simulink library "inp_BCKP"  (R2021b)
settings: Solver=VariableStepAuto  StartTime=0.0  StopTime=10.0  RelTol=1e-3
undefined symbols (not defined in the file): C_TASK_5MS_S, FALSE, KINP_AcoreReadyToSlp_flg_ovrdflg, KINP_AcoreReadyToSlp_flg_ovrdval, KINP_AllowMovThd_OTA_enum_ovrdflg, KINP_AllowMovThd_OTA_enum_ovrdval, KINP_APSAngleTarget_Deg_ovrdflg, KINP_APSAngleTarget_Deg_ovrdval, KINP_APSDecReq_mps2_ovrdflg, KINP_APSDecReq_mps2_ovrdval, KINP_APSDecReqA_flg_ovrdflg, KINP_APSDecReqA_flg_ovrdval, KINP_APSDFLL_cm_ovrdflg, KINP_APSDFLL_cm_ovrdval, KINP_APSDFLR_cm_ovrdflg, KINP_APSDFLR_cm_ovrdval, KINP_APSDRLL_cm_ovrdflg, KINP_APSDRLL_cm_ovrdval, KINP_APSDRLR_cm_ovrdflg, KINP_APSDRLR_cm_ovrdval, KINP_APSExitCondition_enum_ovrdflg, KINP_APSExitCondition_enum_ovrdval, KINP_APSHWVer_enum_ovrdflg, KINP_APSHWVer_enum_ovrdval, KINP_APSProgressPCT_pct_ovrdflg, KINP_APSProgressPCT_pct_ovrdval, KINP_APSPwrReq_enum_ovrdflg, KINP_APSPwrReq_enum_ovrdval, KINP_APSReq_enum_ovrdflg, KINP_APSReq_enum_ovrdval, KINP_APSRQDisplay_enum_ovrdflg, KINP_APSRQDisplay_enum_ovrdval, KINP_APSRqEPASCtrl_flg_ovrdflg, KINP_APSRqEPASCtrl_flg_ovrdval, KINP_APSShiftPosnReq_enum_ovrdval, KINP_APSShiftPosnReq_enum_ovrflg, KINP_APSSpeedCMD_kph_ovrdval, KINP_APSSpeedCMD_kph_ovrflg, KINP_APSStaSystem_enum_ovrdflg, KINP_APSStaSystem_enum_ovrdval, KINP_APSSWVer_enum_ovrdflg, KINP_APSSWVer_enum_ovrdval, KINP_APSVMCReqA_flg_ovrdval, KINP_APSVMCReqA_flg_ovrflg, KINP_APSVRqEPASCtrl_flg_ovrdflg, KINP_APSVRqEPASCtrl_flg_ovrdval, KINP_AuxBattVolmV_mV_ovrdflg, KINP_AuxBattVolmV_mV_ovrdval, KINP_BTConnectSta_enum_ovrdflg, KINP_BTConnectSta_enum_ovrdval, KINP_CAASSta_enum_ovrdflg, KINP_CAASSta_enum_ovrdval, KINP_CAASVMCReqA_flg_ovrdval, KINP_CAASVMCReqA_flg_ovrflg, KINP_CAN1BusOff_flg_ovrdflg, KINP_CAN1BusOff_flg_ovrdval, KINP_CAN2BusOff_flg_ovrdflg, KINP_CAN2BusOff_flg_ovrdval, KINP_CAN3BusOff_flg_ovrdflg, KINP_CAN3BusOff_flg_ovrdval ... (+158)
libraries: FVT_lib x144, hcu_lib x1
(part 3 of 8)

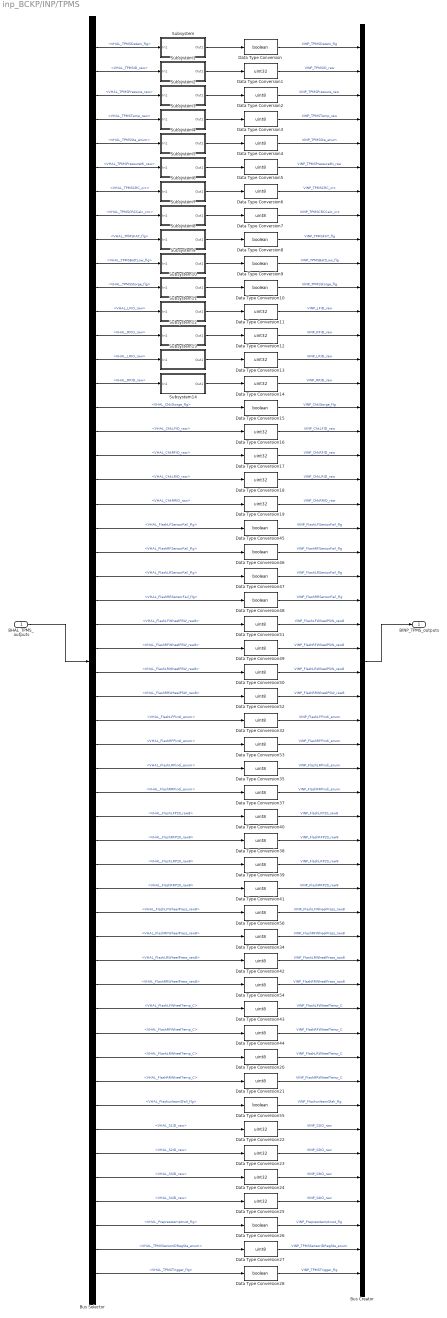
== system inp_BCKP/INP/TPMS ==
  BHAL_TPMS_outputs : Inport  OutDataTypeStr=Bus: BHAL_TPMS_outputs
  Bus Creator : BusCreator  Inputs=52  OutDataTypeStr=Bus: BINP_TPMS_outputs  NonVirtualBus=on
  Bus Selector : BusSelector  OutputSignals=VHAL_TPMSDataIn_flg,VHAL_TPMSID_raw,VHAL_TPMSPressure_raw,VHAL_TPMSTemp_raw,VHAL_TPMSSta_enum,VHAL_TPMSPressureMi_raw,VHAL_TPMSCRC_crc,VHAL_TPMSCRCCalc_crc,VHAL_TPMSFAT_flg,VHAL_TPMSBattLow_flg,VHAL_TPMSStorge_flg,VHAL_LFID_raw,VHAL_RFID_raw,VHAL_LRID_raw,VHAL_RRID_raw,VHAL_ChkStorge_flg,VHAL_ChkLFID_raw,VHAL_ChkRFID_raw,VHAL_ChkLRID_raw,VHAL_ChkRRID_raw,VHAL_FlashLFSensorFail_flg,VHAL_FlashRFSensorFail_flg,VHAL_FlashLRSensorFail_flg,VHAL_FlashRRSensorFail_flg,VHAL_FlashLFWheelPSW_raw8,VHAL_FlashRFWheelPSW_raw8,VHAL_FlashLRWheelPSW_raw8,VHAL_FlashRRWheelPSW_raw8,VHAL_FlashLFPindi_enum,VHAL_FlashRFPindi_enum,VHAL_FlashLRPindi_enum,VHAL_FlashRRPindi_enum,VHAL_FlashLFP20_raw8,VHAL_FlashRFP20_raw8,VHAL_FlashLRP20_raw8,VHAL_FlashRRP20_raw8,VHAL_FlashLFWheelPress_raw8,VHAL_FlashRFWheelPress_raw8,VHAL_FlashLRWheelPress_raw8,VHAL_FlashRRWheelPress_raw8,VHAL_FlashLFWheelTemp_C,VHAL_FlashRFWheelTemp_C,VHAL_FlashLRWheelTemp_C,VHAL_FlashRRWheelTemp_C,VHAL_FlashunlearnSfali_flg,VHAL_S1ID_raw,VHAL_S2ID_raw,VHAL_S3ID_raw,VHAL_S4ID_raw,VHAL_Prepresstemptrust_flg,VHAL_TPMSSensorIDRegSta_enum,VHAL_TPMSTrigger_flg
  Data Type Conversion{,8..10,15,26,28,45..48,55} (12 alike) : DataTypeConversion  OutDataTypeStr=boolean
  Data Type Conversion{1,11..14,16..19,22..25} (13 alike) : DataTypeConversion  OutDataTypeStr=uint32
  Data Type Conversion{2..7,20..21,27,32,34..35,37..44,49..54,56} (27 alike) : DataTypeConversion  OutDataTypeStr=uint8
  Subsystem : Subsystem
  Subsystem1 : Subsystem
  Subsystem10 : Subsystem
  Subsystem11 : Subsystem
  Subsystem12 : Subsystem
  Subsystem13 : Subsystem
  Subsystem14 : Subsystem
  Subsystem2 : Subsystem
  Subsystem3 : Subsystem
  Subsystem4 : Subsystem
  Subsystem5 : Subsystem
  Subsystem6 : Subsystem
  Subsystem7 : Subsystem
  Subsystem8 : Subsystem
  Subsystem9 : Subsystem
  BINP_TPMS_outputs : Outport  OutDataTypeStr=Bus: BINP_TPMS_outputs
  wires:
  Bus Selector/49 -> Data Type Conversion25/1  "<VHAL_S4ID_raw>"
  Bus Selector/48 -> Data Type Conversion24/1  "<VHAL_S3ID_raw>"
  Bus Selector/47 -> Data Type Conversion23/1  "<VHAL_S2ID_raw>"
  Bus Selector/46 -> Data Type Conversion22/1  "<VHAL_S1ID_raw>"
  Data Type Conversion25/1 -> Bus Creator/49  "VINP_S4ID_raw"
  Data Type Conversion24/1 -> Bus Creator/48  "VINP_S3ID_raw"
  Data Type Conversion23/1 -> Bus Creator/47  "VINP_S2ID_raw"
  Data Type Conversion22/1 -> Bus Creator/46  "VINP_S1ID_raw"
  Data Type Conversion21/1 -> Bus Creator/44  "VINP_FlashRRWheelTemp_C"
  Data Type Conversion20/1 -> Bus Creator/43  "VINP_FlashLRWheelTemp_C"
  Bus Selector/44 -> Data Type Conversion21/1  "<VHAL_FlashRRWheelTemp_C>"
  Bus Selector/43 -> Data Type Conversion20/1  "<VHAL_FlashLRWheelTemp_C>"
  Data Type Conversion55/1 -> Bus Creator/45  "VINP_FlashunlearnSfali_flg"
  Bus Selector/45 -> Data Type Conversion55/1  "<VHAL_FlashunlearnSfali_flg>"
  Data Type Conversion44/1 -> Bus Creator/42  "VINP_FlashRFWheelTemp_C"
  Bus Selector/42 -> Data Type Conversion44/1  "<VHAL_FlashRFWheelTemp_C>"
  Data Type Conversion43/1 -> Bus Creator/41  "VINP_FlashLFWheelTemp_C"
  Bus Selector/41 -> Data Type Conversion43/1  "<VHAL_FlashLFWheelTemp_C>"
  Data Type Conversion54/1 -> Bus Creator/40  "VINP_FlashRRWheelPress_raw8"
  Data Type Conversion42/1 -> Bus Creator/39  "VINP_FlashLRWheelPress_raw8"
  Bus Selector/40 -> Data Type Conversion54/1  "<VHAL_FlashRRWheelPress_raw8>"
  Bus Selector/39 -> Data Type Conversion42/1  "<VHAL_FlashLRWheelPress_raw8>"
  Data Type Conversion34/1 -> Bus Creator/38  "VINP_FlashRFWheelPress_raw8"
  Bus Selector/38 -> Data Type Conversion34/1  "<VHAL_FlashRFWheelPress_raw8>"
  Data Type Conversion56/1 -> Bus Creator/37  "VINP_FlashLFWheelPress_raw8"
  Bus Selector/37 -> Data Type Conversion56/1  "<VHAL_FlashLFWheelPress_raw8>"
  Data Type Conversion41/1 -> Bus Creator/36  "VINP_FlashRRP20_raw8"
  Bus Selector/36 -> Data Type Conversion41/1  "<VHAL_FlashRRP20_raw8>"
  Data Type Conversion39/1 -> Bus Creator/35  "VINP_FlashLRP20_raw8"
  Bus Selector/35 -> Data Type Conversion39/1  "<VHAL_FlashLRP20_raw8>"
  Data Type Conversion38/1 -> Bus Creator/34  "VINP_FlashRFP20_raw8"
  Bus Selector/34 -> Data Type Conversion38/1  "<VHAL_FlashRFP20_raw8>"
  Data Type Conversion40/1 -> Bus Creator/33  "VINP_FlashLFP20_raw8"
  Bus Selector/33 -> Data Type Conversion40/1  "<VHAL_FlashLFP20_raw8>"
  Data Type Conversion37/1 -> Bus Creator/32  "VINP_FlashRRPindi_enum"
  Bus Selector/32 -> Data Type Conversion37/1  "<VHAL_FlashRRPindi_enum>"
  Data Type Conversion35/1 -> Bus Creator/31  "VINP_FlashLRPindi_enum"
  Bus Selector/31 -> Data Type Conversion35/1  "<VHAL_FlashLRPindi_enum>"
  Data Type Conversion53/1 -> Bus Creator/30  "VINP_FlashRFPindi_enum"
  Bus Selector/30 -> Data Type Conversion53/1  "<VHAL_FlashRFPindi_enum>"
  Data Type Conversion32/1 -> Bus Creator/29  "VINP_FlashLFPindi_enum"
  Bus Selector/29 -> Data Type Conversion32/1  "<VHAL_FlashLFPindi_enum>"
  Data Type Conversion52/1 -> Bus Creator/28  "VINP_FlashRRWheelPSW_raw8"
  Bus Selector/28 -> Data Type Conversion52/1  "<VHAL_FlashRRWheelPSW_raw8>"
  Data Type Conversion50/1 -> Bus Creator/27  "VINP_FlashLRWheelPSW_raw8"
  Bus Selector/27 -> Data Type Conversion50/1  "<VHAL_FlashLRWheelPSW_raw8>"
  Data Type Conversion49/1 -> Bus Creator/26  "VINP_FlashRFWheelPSW_raw8"
  Bus Selector/26 -> Data Type Conversion49/1  "<VHAL_FlashRFWheelPSW_raw8>"
  Data Type Conversion51/1 -> Bus Creator/25  "VINP_FlashLFWheelPSW_raw8"
  Bus Selector/25 -> Data Type Conversion51/1  "<VHAL_FlashLFWheelPSW_raw8>"
  Data Type Conversion48/1 -> Bus Creator/24  "VINP_FlashRRSensorFail_flg"
  Bus Selector/24 -> Data Type Conversion48/1  "<VHAL_FlashRRSensorFail_flg>"
  Data Type Conversion47/1 -> Bus Creator/23  "VINP_FlashLRSensorFail_flg"
  Bus Selector/23 -> Data Type Conversion47/1  "<VHAL_FlashLRSensorFail_flg>"
  Data Type Conversion46/1 -> Bus Creator/22  "VINP_FlashRFSensorFail_flg"
  Bus Selector/22 -> Data Type Conversion46/1  "<VHAL_FlashRFSensorFail_flg>"
  Data Type Conversion45/1 -> Bus Creator/21  "VINP_FlashLFSensorFail_flg"
  Bus Selector/21 -> Data Type Conversion45/1  "<VHAL_FlashLFSensorFail_flg>"
  Data Type Conversion19/1 -> Bus Creator/20  "VINP_ChkRRID_raw"
  Data Type Conversion18/1 -> Bus Creator/19  "VINP_ChkLRID_raw"
  Data Type Conversion17/1 -> Bus Creator/18  "VINP_ChkRFID_raw"
  Data Type Conversion16/1 -> Bus Creator/17  "VINP_ChkLFID_raw"
  Data Type Conversion15/1 -> Bus Creator/16  "VINP_ChkStorge_flg"
  Bus Selector/20 -> Data Type Conversion19/1  "<VHAL_ChkRRID_raw>"
  Bus Selector/19 -> Data Type Conversion18/1  "<VHAL_ChkLRID_raw>"
  Bus Selector/18 -> Data Type Conversion17/1  "<VHAL_ChkRFID_raw>"
  Bus Selector/17 -> Data Type Conversion16/1  "<VHAL_ChkLFID_raw>"
  Bus Selector/16 -> Data Type Conversion15/1  "<VHAL_ChkStorge_flg>"
  Data Type Conversion14/1 -> Bus Creator/15  "VINP_RRID_raw"
  Data Type Conversion13/1 -> Bus Creator/14  "VINP_LRID_raw"
  Data Type Conversion12/1 -> Bus Creator/13  "VINP_RFID_raw"
  Data Type Conversion11/1 -> Bus Creator/12  "VINP_LFID_raw"
  Subsystem14/1(Out1) -> Data Type Conversion14/1
  Subsystem13/1(Out1) -> Data Type Conversion13/1
  Subsystem12/1(Out1) -> Data Type Conversion12/1
  Subsystem11/1(Out1) -> Data Type Conversion11/1
  Bus Selector/15 -> Subsystem14/1(In1)  "<VHAL_RRID_raw>"
  Bus Selector/14 -> Subsystem13/1(In1)  "<VHAL_LRID_raw>"
  Bus Selector/13 -> Subsystem12/1(In1)  "<VHAL_RFID_raw>"
  Bus Selector/12 -> Subsystem11/1(In1)  "<VHAL_LFID_raw>"
  Data Type Conversion10/1 -> Bus Creator/11  "VINP_TPMSStorge_flg"
  Subsystem10/1(Out1) -> Data Type Conversion10/1
  Bus Selector/11 -> Subsystem10/1(In1)  "<VHAL_TPMSStorge_flg>"
  Subsystem9/1(Out1) -> Data Type Conversion9/1
  Subsystem8/1(Out1) -> Data Type Conversion8/1
  Bus Selector/10 -> Subsystem9/1(In1)  "<VHAL_TPMSBattLow_flg>"
  Bus Selector/9 -> Subsystem8/1(In1)  "<VHAL_TPMSFAT_flg>"
  Data Type Conversion9/1 -> Bus Creator/10  "VINP_TPMSBattLow_flg"
  Data Type Conversion8/1 -> Bus Creator/9  "VINP_TPMSFAT_flg"
  Bus Creator/1 -> BINP_TPMS_outputs/1
  Data Type Conversion7/1 -> Bus Creator/8  "VINP_TPMSCRCCalc_crc"
  Data Type Conversion6/1 -> Bus Creator/7  "VINP_TPMSCRC_crc"
  Data Type Conversion5/1 -> Bus Creator/6  "VINP_TPMSPressureMi_raw"
  Data Type Conversion4/1 -> Bus Creator/5  "VINP_TPMSSta_enum"
  Data Type Conversion3/1 -> Bus Creator/4  "VINP_TPMSTemp_raw"
  Data Type Conversion2/1 -> Bus Creator/3  "VINP_TPMSPressure_raw"
  Data Type Conversion1/1 -> Bus Creator/2  "VINP_TPMSID_raw"
  Data Type Conversion/1 -> Bus Creator/1  "VINP_TPMSDataIn_flg"
  Subsystem7/1(Out1) -> Data Type Conversion7/1
  Subsystem6/1(Out1) -> Data Type Conversion6/1
  Subsystem5/1(Out1) -> Data Type Conversion5/1
  Subsystem4/1(Out1) -> Data Type Conversion4/1
  Subsystem3/1(Out1) -> Data Type Conversion3/1
  Subsystem2/1(Out1) -> Data Type Conversion2/1
  Subsystem1/1(Out1) -> Data Type Conversion1/1
  Subsystem/1(Out1) -> Data Type Conversion/1
  Bus Selector/8 -> Subsystem7/1(In1)  "<VHAL_TPMSCRCCalc_crc>"
  Bus Selector/7 -> Subsystem6/1(In1)  "<VHAL_TPMSCRC_crc>"
  Bus Selector/6 -> Subsystem5/1(In1)  "<VHAL_TPMSPressureMi_raw>"
  Bus Selector/5 -> Subsystem4/1(In1)  "<VHAL_TPMSSta_enum>"
  Bus Selector/4 -> Subsystem3/1(In1)  "<VHAL_TPMSTemp_raw>"
  Bus Selector/3 -> Subsystem2/1(In1)  "<VHAL_TPMSPressure_raw>"
  Bus Selector/2 -> Subsystem1/1(In1)  "<VHAL_TPMSID_raw>"
  Bus Selector/1 -> Subsystem/1(In1)  "<VHAL_TPMSDataIn_flg>"
  BHAL_TPMS_outputs/1 -> Bus Selector/1
  Bus Selector/50 -> Data Type Conversion26/1  "<VHAL_Prepresstemptrust_flg>"
  Data Type Conversion26/1 -> Bus Creator/50  "VINP_Prepresstemptrust_flg"
  Bus Selector/51 -> Data Type Conversion27/1  "<VHAL_TPMSSensorIDRegSta_enum>"
  Data Type Conversion27/1 -> Bus Creator/51  "VINP_TPMSSensorIDRegSta_enum"
  Bus Selector/52 -> Data Type Conversion28/1  "<VHAL_TPMSTrigger_flg>"
  Data Type Conversion28/1 -> Bus Creator/52  "VINP_TPMSTrigger_flg"

== system inp_BCKP/INP/APM/Subsystem ==
  In1 : Inport
  Constant : Constant  Value=KINP_PASDRMR_cm_ovrdval
  Constant1 : Constant  Value=KINP_PASDRMR_cm_ovrdflg
  Switch : Switch  Criteria=u2 ~= 0
  Out1 : Outport
  wires:
  Switch/1 -> Out1/1
  In1/1 -> Switch/3
  Constant/1 -> Switch/1
  Constant1/1 -> Switch/2

== system inp_BCKP/INP/APM/Subsystem1 ==
  In1 : Inport
  Constant : Constant  Value=KINP_PASDRML_cm_ovrdval
  Constant1 : Constant  Value=KINP_PASDRML_cm_ovrdflg
  Switch : Switch  Criteria=u2 ~= 0
  Out1 : Outport
  wires:
  Constant1/1 -> Switch/2
  Constant/1 -> Switch/1
  In1/1 -> Switch/3
  Switch/1 -> Out1/1

== system inp_BCKP/INP/APM/Subsystem10 ==
  In1 : Inport
  Constant : Constant  Value=KINP_APSDFLR_cm_ovrdval
  Constant1 : Constant  Value=KINP_APSDFLR_cm_ovrdflg
  Switch : Switch  Criteria=u2 ~= 0
  Out1 : Outport
  wires:
  Switch/1 -> Out1/1
  In1/1 -> Switch/3
  Constant/1 -> Switch/1
  Constant1/1 -> Switch/2

== system inp_BCKP/INP/APM/Subsystem11 ==
  In1 : Inport
  Constant : Constant  Value=KINP_APSDFLL_cm_ovrdval
  Constant1 : Constant  Value=KINP_APSDFLL_cm_ovrdflg
  Switch : Switch  Criteria=u2 ~= 0
  Out1 : Outport
  wires:
  Constant1/1 -> Switch/2
  Constant/1 -> Switch/1
  In1/1 -> Switch/3
  Switch/1 -> Out1/1

== system inp_BCKP/INP/APM/Subsystem12 ==
  In1 : Inport
  Constant : Constant  Value=KINP_PASAFCL_enum_ovrdval
  Constant1 : Constant  Value=KINP_PASAFCL_enum_ovrdflg
  Switch : Switch  Criteria=u2 ~= 0
  Out1 : Outport
  wires:
  Switch/1 -> Out1/1
  In1/1 -> Switch/3
  Constant/1 -> Switch/1
  Constant1/1 -> Switch/2

== system inp_BCKP/INP/APM/Subsystem13 ==
  In1 : Inport
  Constant : Constant  Value=KINP_PASARMR_enum_ovrdval
  Constant1 : Constant  Value=KINP_PASARMR_enum_ovrdflg
  Switch : Switch  Criteria=u2 ~= 0
  Out1 : Outport
  wires:
  Constant1/1 -> Switch/2
  Constant/1 -> Switch/1
  In1/1 -> Switch/3
  Switch/1 -> Out1/1

== system inp_BCKP/INP/APM/Subsystem14 ==
  In1 : Inport
  Constant : Constant  Value=KINP_PASARML_enum_ovrdval
  Constant1 : Constant  Value=KINP_PASARML_enum_ovrdflg
  Switch : Switch  Criteria=u2 ~= 0
  Out1 : Outport
  wires:
  Switch/1 -> Out1/1
  In1/1 -> Switch/3
  Constant/1 -> Switch/1
  Constant1/1 -> Switch/2

== system inp_BCKP/INP/APM/Subsystem15 ==
  In1 : Inport
  Constant : Constant  Value=KINP_PASARCR_enum_ovrdval
  Constant1 : Constant  Value=KINP_PASARCR_enum_ovrdflg
  Switch : Switch  Criteria=u2 ~= 0
  Out1 : Outport
  wires:
  Constant1/1 -> Switch/2
  Constant/1 -> Switch/1
  In1/1 -> Switch/3
  Switch/1 -> Out1/1

== system inp_BCKP/INP/APM/Subsystem16 ==
  In1 : Inport
  Constant : Constant  Value=KINP_PASARCL_enum_ovrdval
  Constant1 : Constant  Value=KINP_PASARCL_enum_ovrdflg
  Switch : Switch  Criteria=u2 ~= 0
  Out1 : Outport
  wires:
  Switch/1 -> Out1/1
  In1/1 -> Switch/3
  Constant/1 -> Switch/1
  Constant1/1 -> Switch/2

== system inp_BCKP/INP/APM/Subsystem17 ==
  In1 : Inport
  Constant : Constant  Value=KINP_PASAFMR_enum_ovrdval
  Constant1 : Constant  Value=KINP_PASAFMR_enum_ovrdflg
  Switch : Switch  Criteria=u2 ~= 0
  Out1 : Outport
  wires:
  Constant1/1 -> Switch/2
  Constant/1 -> Switch/1
  In1/1 -> Switch/3
  Switch/1 -> Out1/1

== system inp_BCKP/INP/APM/Subsystem18 ==
  In1 : Inport
  Constant : Constant  Value=KINP_PASAFML_enum_ovrdval
  Constant1 : Constant  Value=KINP_PASAFML_enum_ovrdflg
  Switch : Switch  Criteria=u2 ~= 0
  Out1 : Outport
  wires:
  Switch/1 -> Out1/1
  In1/1 -> Switch/3
  Constant/1 -> Switch/1
  Constant1/1 -> Switch/2

== system inp_BCKP/INP/APM/Subsystem19 ==
  In1 : Inport
  Constant : Constant  Value=KINP_PASAFCR_enum_ovrdval
  Constant1 : Constant  Value=KINP_PASAFCR_enum_ovrdflg
  Switch : Switch  Criteria=u2 ~= 0
  Out1 : Outport
  wires:
  Constant1/1 -> Switch/2
  Constant/1 -> Switch/1
  In1/1 -> Switch/3
  Switch/1 -> Out1/1

== system inp_BCKP/INP/APM/Subsystem2 ==
  In1 : Inport
  Constant : Constant  Value=KINP_PASDRCR_cm_ovrdval
  Constant1 : Constant  Value=KINP_PASDRCR_cm_ovrdflg
  Switch : Switch  Criteria=u2 ~= 0
  Out1 : Outport
  wires:
  Constant1/1 -> Switch/2
  Constant/1 -> Switch/1
  In1/1 -> Switch/3
  Switch/1 -> Out1/1

== system inp_BCKP/INP/APM/Subsystem20 ==
  In1 : Inport
  Constant : Constant  Value=KINP_USSStaRMR_flg_ovrdval
  Constant1 : Constant  Value=KINP_USSStaRMR_flg_ovrdflg
  Switch : Switch  Criteria=u2 ~= 0
  Out1 : Outport
  wires:
  Switch/1 -> Out1/1
  In1/1 -> Switch/3
  Constant/1 -> Switch/1
  Constant1/1 -> Switch/2

== system inp_BCKP/INP/APM/Subsystem21 ==
  In1 : Inport
  Constant : Constant  Value=KINP_USSStaRML_flg_ovrdval
  Constant1 : Constant  Value=KINP_USSStaRML_flg_ovrdflg
  Switch : Switch  Criteria=u2 ~= 0
  Out1 : Outport
  wires:
  Constant1/1 -> Switch/2
  Constant/1 -> Switch/1
  In1/1 -> Switch/3
  Switch/1 -> Out1/1

== system inp_BCKP/INP/APM/Subsystem22 ==
  In1 : Inport
  Constant : Constant  Value=KINP_USSStaRLR_flg_ovrdval
  Constant1 : Constant  Value=KINP_USSStaRLR_flg_ovrdflg
  Switch : Switch  Criteria=u2 ~= 0
  Out1 : Outport
  wires:
  Switch/1 -> Out1/1
  In1/1 -> Switch/3
  Constant/1 -> Switch/1
  Constant1/1 -> Switch/2

== system inp_BCKP/INP/APM/Subsystem23 ==
  In1 : Inport
  Constant : Constant  Value=KINP_USSStaRLL_flg_ovrdval
  Constant1 : Constant  Value=KINP_USSStaRLL_flg_ovrdflg
  Switch : Switch  Criteria=u2 ~= 0
  Out1 : Outport
  wires:
  Constant1/1 -> Switch/2
  Constant/1 -> Switch/1
  In1/1 -> Switch/3
  Switch/1 -> Out1/1

== system inp_BCKP/INP/APM/Subsystem24 ==
  In1 : Inport
  Constant : Constant  Value=KINP_USSStaRCR_flg_ovrdval
  Constant1 : Constant  Value=KINP_USSStaRCR_flg_ovrdflg
  Switch : Switch  Criteria=u2 ~= 0
  Out1 : Outport
  wires:
  Switch/1 -> Out1/1
  In1/1 -> Switch/3
  Constant/1 -> Switch/1
  Constant1/1 -> Switch/2

== system inp_BCKP/INP/APM/Subsystem25 ==
  In1 : Inport
  Constant : Constant  Value=KINP_USSStaRCL_flg_ovrdval
  Constant1 : Constant  Value=KINP_USSStaRCL_flg_ovrdflg
  Switch : Switch  Criteria=u2 ~= 0
  Out1 : Outport
  wires:
  Constant1/1 -> Switch/2
  Constant/1 -> Switch/1
  In1/1 -> Switch/3
  Switch/1 -> Out1/1

== system inp_BCKP/INP/APM/Subsystem26 ==
  In1 : Inport
  Constant : Constant  Value=KINP_USSStaFMR_flg_ovrdval
  Constant1 : Constant  Value=KINP_USSStaFMR_flg_ovrdflg
  Switch : Switch  Criteria=u2 ~= 0
  Out1 : Outport
  wires:
  Switch/1 -> Out1/1
  In1/1 -> Switch/3
  Constant/1 -> Switch/1
  Constant1/1 -> Switch/2

== system inp_BCKP/INP/APM/Subsystem27 ==
  In1 : Inport
  Constant : Constant  Value=KINP_USSStaFML_flg_ovrdval
  Constant1 : Constant  Value=KINP_USSStaFML_flg_ovrdflg
  Switch : Switch  Criteria=u2 ~= 0
  Out1 : Outport
  wires:
  Constant1/1 -> Switch/2
  Constant/1 -> Switch/1
  In1/1 -> Switch/3
  Switch/1 -> Out1/1

== system inp_BCKP/INP/APM/Subsystem28 ==
  In1 : Inport
  Constant : Constant  Value=KINP_USSStaFLR_flg_ovrdval
  Constant1 : Constant  Value=KINP_USSStaFLR_flg_ovrdflg
  Switch : Switch  Criteria=u2 ~= 0
  Out1 : Outport
  wires:
  Switch/1 -> Out1/1
  In1/1 -> Switch/3
  Constant/1 -> Switch/1
  Constant1/1 -> Switch/2

== system inp_BCKP/INP/APM/Subsystem29 ==
  In1 : Inport
  Constant : Constant  Value=KINP_USSStaFLL_flg_ovrdval
  Constant1 : Constant  Value=KINP_USSStaFLL_flg_ovrdflg
  Switch : Switch  Criteria=u2 ~= 0
  Out1 : Outport
  wires:
  Constant1/1 -> Switch/2
  Constant/1 -> Switch/1
  In1/1 -> Switch/3
  Switch/1 -> Out1/1

== system inp_BCKP/INP/APM/Subsystem3 ==
  In1 : Inport
  Constant : Constant  Value=KINP_PASDRCL_cm_ovrdval
  Constant1 : Constant  Value=KINP_PASDRCL_cm_ovrdflg
  Switch : Switch  Criteria=u2 ~= 0
  Out1 : Outport
  wires:
  Constant1/1 -> Switch/2
  Constant/1 -> Switch/1
  In1/1 -> Switch/3
  Switch/1 -> Out1/1

== system inp_BCKP/INP/APM/Subsystem30 ==
  In1 : Inport
  Constant : Constant  Value=KINP_USSStaFCR_flg_ovrdval
  Constant1 : Constant  Value=KINP_USSStaFCR_flg_ovrdflg
  Switch : Switch  Criteria=u2 ~= 0
  Out1 : Outport
  wires:
  Switch/1 -> Out1/1
  In1/1 -> Switch/3
  Constant/1 -> Switch/1
  Constant1/1 -> Switch/2

== system inp_BCKP/INP/APM/Subsystem31 ==
  In1 : Inport
  Constant : Constant  Value=KINP_USSStaFCL_flg_ovrdval
  Constant1 : Constant  Value=KINP_USSStaFCL_flg_ovrdflg
  Switch : Switch  Criteria=u2 ~= 0
  Out1 : Outport
  wires:
  Constant1/1 -> Switch/2
  Constant/1 -> Switch/1
  In1/1 -> Switch/3
  Switch/1 -> Out1/1

== system inp_BCKP/INP/APM/Subsystem32 ==
  In1 : Inport
  Constant : Constant  Value=KINP_Chime_enum_ovrdval
  Constant1 : Constant  Value=KINP_Chime_enum_ovrdflg
  Switch : Switch  Criteria=u2 ~= 0
  Out1 : Outport
  wires:
  Switch/1 -> Out1/1
  In1/1 -> Switch/3
  Constant/1 -> Switch/1
  Constant1/1 -> Switch/2

== system inp_BCKP/INP/APM/Subsystem33 ==
  In1 : Inport
  Constant : Constant  Value=KINP_SNSRLayout_enum_ovrdval
  Constant1 : Constant  Value=KINP_SNSRLayout_enum_ovrdflg
  Switch : Switch  Criteria=u2 ~= 0
  Out1 : Outport
  wires:
  Constant1/1 -> Switch/2
  Constant/1 -> Switch/1
  In1/1 -> Switch/3
  Switch/1 -> Out1/1

== system inp_BCKP/INP/APM/Subsystem34 ==
  In1 : Inport
  Constant : Constant  Value=KINP_StaFSya_flg_ovrdval
  Constant1 : Constant  Value=KINP_StaFSya_flg_ovrdflg
  Switch : Switch  Criteria=u2 ~= 0
  Out1 : Outport
  wires:
  Switch/1 -> Out1/1
  In1/1 -> Switch/3
  Constant/1 -> Switch/1
  Constant1/1 -> Switch/2

== system inp_BCKP/INP/APM/Subsystem35 ==
  In1 : Inport
  Constant : Constant  Value=KINP_ModOperation_enum_ovrdval
  Constant1 : Constant  Value=KINP_ModOperation_enum_ovrdflg
  Switch : Switch  Criteria=u2 ~= 0
  Out1 : Outport
  wires:
  Constant1/1 -> Switch/2
  Constant/1 -> Switch/1
  In1/1 -> Switch/3
  Switch/1 -> Out1/1

== system inp_BCKP/INP/APM/Subsystem36 ==
  In1 : Inport
  Constant : Constant  Value=KINP_APSVMCReqA_flg_ovrflg
  Constant1 : Constant  Value=KINP_APSVMCReqA_flg_ovrdval
  Switch : Switch  Criteria=u2 ~= 0
  Out1 : Outport
  wires:
  Constant/1 -> Switch/2
  Constant1/1 -> Switch/1
  In1/1 -> Switch/3
  Switch/1 -> Out1/1

== system inp_BCKP/INP/APM/Subsystem37 ==
  In1 : Inport
  Constant : Constant  Value=KINP_APSShiftPosnReq_enum_ovrflg
  Constant1 : Constant  Value=KINP_APSShiftPosnReq_enum_ovrdval
  Switch : Switch  Criteria=u2 ~= 0
  Out1 : Outport
  wires:
  Switch/1 -> Out1/1
  In1/1 -> Switch/3
  Constant1/1 -> Switch/1
  Constant/1 -> Switch/2

== system inp_BCKP/INP/APM/Subsystem38 ==
  In1 : Inport
  Constant : Constant  Value=KINP_APSSpeedCMD_kph_ovrflg
  Constant1 : Constant  Value=KINP_APSSpeedCMD_kph_ovrdval
  Switch : Switch  Criteria=u2 ~= 0
  Out1 : Outport
  wires:
  Constant/1 -> Switch/2
  Constant1/1 -> Switch/1
  In1/1 -> Switch/3
  Switch/1 -> Out1/1

== system inp_BCKP/INP/APM/Subsystem39 ==
  In1 : Inport
  Constant : Constant  Value=KINP_CAASVMCReqA_flg_ovrflg
  Constant1 : Constant  Value=KINP_CAASVMCReqA_flg_ovrdval
  Switch : Switch  Criteria=u2 ~= 0
  Out1 : Outport
  wires:
  Switch/1 -> Out1/1
  In1/1 -> Switch/3
  Constant1/1 -> Switch/1
  Constant/1 -> Switch/2

== system inp_BCKP/INP/APM/Subsystem4 ==
  In1 : Inport
  Constant : Constant  Value=KINP_PASDFMR_cm_ovrdval
  Constant1 : Constant  Value=KINP_PASDFMR_cm_ovrdflg
  Switch : Switch  Criteria=u2 ~= 0
  Out1 : Outport
  wires:
  Switch/1 -> Out1/1
  In1/1 -> Switch/3
  Constant/1 -> Switch/1
  Constant1/1 -> Switch/2

== system inp_BCKP/INP/APM/Subsystem40 ==
  In1 : Inport
  Constant : Constant  Value=KINP_APSProgressPCT_pct_ovrdval
  Constant1 : Constant  Value=KINP_APSProgressPCT_pct_ovrdflg
  Switch : Switch  Criteria=u2 ~= 0
  Out1 : Outport
  wires:
  Switch/1 -> Out1/1
  In1/1 -> Switch/3
  Constant/1 -> Switch/1
  Constant1/1 -> Switch/2

== system inp_BCKP/INP/APM/Subsystem41 ==
  In1 : Inport
  Constant : Constant  Value=KINP_APSRQDisplay_enum_ovrdval
  Constant1 : Constant  Value=KINP_APSRQDisplay_enum_ovrdflg
  Switch : Switch  Criteria=u2 ~= 0
  Out1 : Outport
  wires:
  Switch/1 -> Out1/1
  In1/1 -> Switch/3
  Constant/1 -> Switch/1
  Constant1/1 -> Switch/2

== system inp_BCKP/INP/APM/Subsystem42 ==
  In1 : Inport
  Constant : Constant  Value=KINP_APSSWVer_enum_ovrdval
  Constant1 : Constant  Value=KINP_APSSWVer_enum_ovrdflg
  Switch : Switch  Criteria=u2 ~= 0
  Out1 : Outport
  wires:
  Switch/1 -> Out1/1
  In1/1 -> Switch/3
  Constant/1 -> Switch/1
  Constant1/1 -> Switch/2

== system inp_BCKP/INP/APM/Subsystem43 ==
  In1 : Inport
  Constant : Constant  Value=KINP_APSHWVer_enum_ovrdval
  Constant1 : Constant  Value=KINP_APSHWVer_enum_ovrdflg
  Switch : Switch  Criteria=u2 ~= 0
  Out1 : Outport
  wires:
  Switch/1 -> Out1/1
  In1/1 -> Switch/3
  Constant/1 -> Switch/1
  Constant1/1 -> Switch/2

== system inp_BCKP/INP/APM/Subsystem44 ==
  In1 : Inport
  Constant : Constant  Value=KINP_APSExitCondition_enum_ovrdval
  Constant1 : Constant  Value=KINP_APSExitCondition_enum_ovrdflg
  Switch : Switch  Criteria=u2 ~= 0
  Out1 : Outport
  wires:
  Switch/1 -> Out1/1
  In1/1 -> Switch/3
  Constant/1 -> Switch/1
  Constant1/1 -> Switch/2

== system inp_BCKP/INP/APM/Subsystem45 ==
  In1 : Inport
  Constant : Constant  Value=KINP_APSAngleTarget_Deg_ovrdval
  Constant1 : Constant  Value=KINP_APSAngleTarget_Deg_ovrdflg
  Switch : Switch  Criteria=u2 ~= 0
  Out1 : Outport
  wires:
  Switch/1 -> Out1/1
  In1/1 -> Switch/3
  Constant/1 -> Switch/1
  Constant1/1 -> Switch/2

== system inp_BCKP/INP/APM/Subsystem46 ==
  In1 : Inport
  Constant : Constant  Value=KINP_APSStaSystem_enum_ovrdval
  Constant1 : Constant  Value=KINP_APSStaSystem_enum_ovrdflg
  Switch : Switch  Criteria=u2 ~= 0
  Out1 : Outport
  wires:
  Switch/1 -> Out1/1
  In1/1 -> Switch/3
  Constant/1 -> Switch/1
  Constant1/1 -> Switch/2

== system inp_BCKP/INP/APM/Subsystem47 ==
  In1 : Inport
  Constant : Constant  Value=KINP_APSVRqEPASCtrl_flg_ovrdval
  Constant1 : Constant  Value=KINP_APSVRqEPASCtrl_flg_ovrdflg
  Switch : Switch  Criteria=u2 ~= 0
  Out1 : Outport
  wires:
  Constant1/1 -> Switch/2
  Constant/1 -> Switch/1
  In1/1 -> Switch/3
  Switch/1 -> Out1/1

== system inp_BCKP/INP/APM/Subsystem48 ==
  In1 : Inport
  Constant : Constant  Value=KINP_APSRqEPASCtrl_flg_ovrdval
  Constant1 : Constant  Value=KINP_APSRqEPASCtrl_flg_ovrdflg
  Switch : Switch  Criteria=u2 ~= 0
  Out1 : Outport
  wires:
  Switch/1 -> Out1/1
  In1/1 -> Switch/3
  Constant/1 -> Switch/1
  Constant1/1 -> Switch/2

== system inp_BCKP/INP/APM/Subsystem49 ==
  In1 : Inport
  Constant : Constant  Value=KINP_APSReq_enum_ovrdval
  Constant1 : Constant  Value=KINP_APSReq_enum_ovrdflg
  Switch : Switch  Criteria=u2 ~= 0
  Out1 : Outport
  wires:
  Constant1/1 -> Switch/2
  Constant/1 -> Switch/1
  In1/1 -> Switch/3
  Switch/1 -> Out1/1

== system inp_BCKP/INP/APM/Subsystem5 ==
  In1 : Inport
  Constant : Constant  Value=KINP_PASDFML_cm_ovrdval
  Constant1 : Constant  Value=KINP_PASDFML_cm_ovrdflg
  Switch : Switch  Criteria=u2 ~= 0
  Out1 : Outport
  wires:
  Constant1/1 -> Switch/2
  Constant/1 -> Switch/1
  In1/1 -> Switch/3
  Switch/1 -> Out1/1

== system inp_BCKP/INP/APM/Subsystem50 ==
  In1 : Inport
  Constant : Constant  Value=KINP_APSDecReq_mps2_ovrdval
  Constant1 : Constant  Value=KINP_APSDecReq_mps2_ovrdflg
  Switch : Switch  Criteria=u2 ~= 0
  Out1 : Outport
  wires:
  Constant1/1 -> Switch/2
  Constant/1 -> Switch/1
  In1/1 -> Switch/3
  Switch/1 -> Out1/1

== system inp_BCKP/INP/APM/Subsystem51 ==
  In1 : Inport
  Constant : Constant  Value=KINP_APSDecReqA_flg_ovrdval
  Constant1 : Constant  Value=KINP_APSDecReqA_flg_ovrdflg
  Switch : Switch  Criteria=u2 ~= 0
  Out1 : Outport
  wires:
  Constant1/1 -> Switch/2
  Constant/1 -> Switch/1
  In1/1 -> Switch/3
  Switch/1 -> Out1/1

== system inp_BCKP/INP/APM/Subsystem52 ==
  In1 : Inport
  Constant : Constant  Value=KINP_CAASSta_enum_ovrdval
  Constant1 : Constant  Value=KINP_CAASSta_enum_ovrdflg
  Switch : Switch  Criteria=u2 ~= 0
  Out1 : Outport
  wires:
  Constant1/1 -> Switch/2
  Constant/1 -> Switch/1
  In1/1 -> Switch/3
  Switch/1 -> Out1/1

== system inp_BCKP/INP/APM/Subsystem53 ==
  In1 : Inport
  Constant : Constant  Value=KINP_APSPwrReq_enum_ovrdflg
  Constant1 : Constant  Value=KINP_APSPwrReq_enum_ovrdval
  Switch : Switch  Criteria=u2 ~= 0
  Out1 : Outport
  wires:
  Switch/1 -> Out1/1
  Constant1/1 -> Switch/1
  Constant/1 -> Switch/2
  In1/1 -> Switch/3

== system inp_BCKP/INP/APM/Subsystem54 ==
  In1 : Inport
  Constant : Constant  Value=KINP_RAPSBCMLamp_enum_ovrdflg
  Constant1 : Constant  Value=KINP_RAPSBCMLamp_enum_ovrdval
  Switch : Switch  Criteria=u2 ~= 0
  Out1 : Outport
  wires:
  Constant/1 -> Switch/2
  Constant1/1 -> Switch/1
  In1/1 -> Switch/3
  Switch/1 -> Out1/1

== system inp_BCKP/INP/APM/Subsystem55 ==
  In1 : Inport
  Constant : Constant  Value=KINP_RAPSBCMLockReq_flg_ovrdval
  Constant1 : Constant  Value=KINP_RAPSBCMLockReq_flg_ovrflg
  Switch : Switch  Criteria=u2 ~= 0
  Out1 : Outport
  wires:
  Switch/1 -> Out1/1
  Constant/1 -> Switch/1
  Constant1/1 -> Switch/2
  In1/1 -> Switch/3

== system inp_BCKP/INP/APM/Subsystem56 ==
  In1 : Inport
  Constant : Constant  Value=KINP_RAPSErrLv1_flg_ovrflg
  Constant1 : Constant  Value=KINP_RAPSErrLv1_flg_ovrdval
  Switch : Switch  Criteria=u2 ~= 0
  Out1 : Outport
  wires:
  Switch/1 -> Out1/1
  Constant1/1 -> Switch/1
  Constant/1 -> Switch/2
  In1/1 -> Switch/3

== system inp_BCKP/INP/APM/Subsystem57 ==
  In1 : Inport
  Constant : Constant  Value=KINP_RAPSErrWarnSta_enum_ovrdval
  Constant1 : Constant  Value=KINP_RAPSErrWarnSta_enum_ovrdflg
  Switch : Switch  Criteria=u2 ~= 0
  Out1 : Outport
  wires:
  Constant1/1 -> Switch/2
  Constant/1 -> Switch/1
  Switch/1 -> Out1/1
  In1/1 -> Switch/3

== system inp_BCKP/INP/APM/Subsystem6 ==
  In1 : Inport
  Constant : Constant  Value=KINP_PASDFCR_cm_ovrdval
  Constant1 : Constant  Value=KINP_PASDFCR_cm_ovrdflg
  Switch : Switch  Criteria=u2 ~= 0
  Out1 : Outport
  wires:
  Switch/1 -> Out1/1
  In1/1 -> Switch/3
  Constant/1 -> Switch/1
  Constant1/1 -> Switch/2

== system inp_BCKP/INP/APM/Subsystem7 ==
  In1 : Inport
  Constant : Constant  Value=KINP_PASDFCL_cm_ovrdval
  Constant1 : Constant  Value=KINP_PASDFCL_cm_ovrdflg
  Switch : Switch  Criteria=u2 ~= 0
  Out1 : Outport
  wires:
  Constant1/1 -> Switch/2
  Constant/1 -> Switch/1
  In1/1 -> Switch/3
  Switch/1 -> Out1/1

== system inp_BCKP/INP/APM/Subsystem8 ==
  In1 : Inport
  Constant : Constant  Value=KINP_APSDRLR_cm_ovrdval
  Constant1 : Constant  Value=KINP_APSDRLR_cm_ovrdflg
  Switch : Switch  Criteria=u2 ~= 0
  Out1 : Outport
  wires:
  Switch/1 -> Out1/1
  In1/1 -> Switch/3
  Constant/1 -> Switch/1
  Constant1/1 -> Switch/2

== system inp_BCKP/INP/APM/Subsystem9 ==
  In1 : Inport
  Constant : Constant  Value=KINP_APSDRLL_cm_ovrdval
  Constant1 : Constant  Value=KINP_APSDRLL_cm_ovrdflg
  Switch : Switch  Criteria=u2 ~= 0
  Out1 : Outport
  wires:
  Constant1/1 -> Switch/2
  Constant/1 -> Switch/1
  In1/1 -> Switch/3
  Switch/1 -> Out1/1

== system inp_BCKP/INP/CAN1/CommunicationCheck ==
  BHAL_outputs : Inport
  CANMsgInvalidACBTMSC10000 : FVT_lib/inp/CAN_Msg_Validity_Process_template  SystemSampleTime=-1  VariantActivationTime=update diagram  Latency=0  AutoFrameSizeCalculation=off
      link override ovrdflg: Value=KINP_CANMsgInvalidACBTMSC10000_flg_ovrdflg
      link override ovrdval: Value=KINP_CANMsgInvalidACBTMSC10000_flg_ovrdval
  CANMsgInvalidACBTMSC10001 : FVT_lib/inp/CAN_Msg_Validity_Process_template  SystemSampleTime=-1  VariantActivationTime=update diagram  Latency=0  AutoFrameSizeCalculation=off
      link override ovrdflg: Value=KINP_CANMsgInvalidACBTMSC10001_flg_ovrdflg
      link override ovrdval: Value=KINP_CANMsgInvalidACBTMSC10001_flg_ovrdval
  CANMsgInvalidACBTMSC10004 : FVT_lib/inp/CAN_Msg_Validity_Process_template  SystemSampleTime=-1  VariantActivationTime=update diagram  Latency=0  AutoFrameSizeCalculation=off
      link override ovrdflg: Value=KINP_CANMsgInvalidACBTMSC10004_flg_ovrdflg
      link override ovrdval: Value=KINP_CANMsgInvalidACBTMSC10004_flg_ovrdval
  CANMsgInvalidACBTMSC50000 : FVT_lib/inp/CAN_Msg_Validity_Process_template  SystemSampleTime=-1  VariantActivationTime=update diagram  Latency=0  AutoFrameSizeCalculation=off
      link override ovrdflg: Value=KINP_CANMsgInvalidACBTMSC50000_flg_ovrdflg
      link override ovrdval: Value=KINP_CANMsgInvalidACBTMSC50000_flg_ovrdval
  CANMsgInvalidASC1A : FVT_lib/inp/CAN_Msg_Validity_Process_template  SystemSampleTime=-1  VariantActivationTime=update diagram  Latency=0  AutoFrameSizeCalculation=off
      link override ovrdflg: Value=KINP_CANMsgInvalidASC1A_flg_ovrdflg
      link override ovrdval: Value=KINP_CANMsgInvalidASC1A_flg_ovrdval
  CANMsgInvalidEBC1 : FVT_lib/inp/CAN_Msg_Validity_Process_template  SystemSampleTime=-1  VariantActivationTime=update diagram  Latency=0  AutoFrameSizeCalculation=off
      link override ovrdflg: Value=KINP_CANMsgInvalidEBC1_flg_ovrdflg
      link override ovrdval: Value=KINP_CANMsgInvalidEBC1_flg_ovrdval
  CANMsgInvalidEBC2 : FVT_lib/inp/CAN_Msg_Validity_Process_template  SystemSampleTime=-1  VariantActivationTime=update diagram  Latency=0  AutoFrameSizeCalculation=off
      link override ovrdflg: Value=KINP_CANMsgInvalidEBC2_flg_ovrdflg
      link override ovrdval: Value=KINP_CANMsgInvalidEBC2_flg_ovrdval
  CANMsgInvalidEBC5 : FVT_lib/inp/CAN_Msg_Validity_Process_template  SystemSampleTime=-1  VariantActivationTime=update diagram  Latency=0  AutoFrameSizeCalculation=off
      link override ovrdflg: Value=KINP_CANMsgInvalidEBC5_flg_ovrdflg
      link override ovrdval: Value=KINP_CANMsgInvalidEBC5_flg_ovrdval
  CANMsgInvalidECASDM1 : FVT_lib/inp/CAN_Msg_Validity_Process_template  SystemSampleTime=-1  VariantActivationTime=update diagram  Latency=0  AutoFrameSizeCalculation=off
      link override ovrdflg: Value=KINP_CANMsgInvalidECASDM1_flg_ovrdflg
      link override ovrdval: Value=KINP_CANMsgInvalidECASDM1_flg_ovrdval
  CANMsgInvalidEMC1EM1 : FVT_lib/inp/CAN_Msg_Validity_Process_template  SystemSampleTime=-1  VariantActivationTime=update diagram  Latency=0  AutoFrameSizeCalculation=off
      link override ovrdflg: Value=KINP_CANMsgInvalidEMC1EM1_flg_ovrdflg
      link override ovrdval: Value=KINP_CANMsgInvalidEMC1EM1_flg_ovrdval
  CANMsgInvalidHRW : FVT_lib/inp/CAN_Msg_Validity_Process_template  SystemSampleTime=-1  VariantActivationTime=update diagram  Latency=0  AutoFrameSizeCalculation=off
      link override ovrdflg: Value=KINP_CANMsgInvalidHRW_flg_ovrdflg
      link override ovrdval: Value=KINP_CANMsgInvalidHRW_flg_ovrdval
  CANMsgInvalidTC1 : FVT_lib/inp/CAN_Msg_Validity_Process_template  SystemSampleTime=-1  VariantActivationTime=update diagram  Latency=0  AutoFrameSizeCalculation=off
      link override ovrdflg: Value=KINP_CANMsgInvalidTC1_flg_ovrdflg
      link override ovrdval: Value=KINP_CANMsgInvalidTC1_flg_ovrdval
  bus_creator : BusCreator  Inputs=12
  bus_selector : BusSelector  OutputSignals=VHAL_CANMsgInvalidACBTMSC10000_flg,VHAL_CANMsgInvalidACBTMSC10001_flg,VHAL_CANMsgInvalidACBTMSC10004_flg,VHAL_CANMsgInvalidACBTMSC50000_flg,VHAL_CANMsgInvalidASC1A_flg,VHAL_CANMsgInvalidEBC1_flg,VHAL_CANMsgInvalidEBC2_flg,VHAL_CANMsgInvalidEBC5_flg,VHAL_CANMsgInvalidECASDM1_flg,VHAL_CANMsgInvalidEMC1EM1_flg,VHAL_CANMsgInvalidHRW_flg,VHAL_CANMsgInvalidTC1_flg
  not{1..12} (12 alike) : Logic  Operator=NOT  AllPortsSameDT=off  OutDataTypeStr=boolean
  inp_CanValid_bus : Outport
  wires:
  BHAL_outputs/1 -> [BHAL_outputs]
  bus_selector/1 -> CANMsgInvalidACBTMSC10000/1  "<VHAL_CANMsgInvalidACBTMSC10000_flg>"
  CANMsgInvalidACBTMSC10000/1 -> not1/1
  not1/1 -> bus_creator/1  "VINP_CANMsgValidACBTMSC10000_flg"
  bus_selector/2 -> CANMsgInvalidACBTMSC10001/1  "<VHAL_CANMsgInvalidACBTMSC10001_flg>"
  CANMsgInvalidACBTMSC10001/1 -> not2/1
  not2/1 -> bus_creator/2  "VINP_CANMsgValidACBTMSC10001_flg"
  bus_selector/3 -> CANMsgInvalidACBTMSC10004/1  "<VHAL_CANMsgInvalidACBTMSC10004_flg>"
  CANMsgInvalidACBTMSC10004/1 -> not3/1
  not3/1 -> bus_creator/3  "VINP_CANMsgValidACBTMSC10004_flg"
  bus_selector/4 -> CANMsgInvalidACBTMSC50000/1  "<VHAL_CANMsgInvalidACBTMSC50000_flg>"
  CANMsgInvalidACBTMSC50000/1 -> not4/1
  not4/1 -> bus_creator/4  "VINP_CANMsgValidACBTMSC50000_flg"
  bus_selector/5 -> CANMsgInvalidASC1A/1  "<VHAL_CANMsgInvalidASC1A_flg>"
  CANMsgInvalidASC1A/1 -> not5/1
  not5/1 -> bus_creator/5  "VINP_CANMsgValidASC1A_flg"
  bus_selector/6 -> CANMsgInvalidEBC1/1  "<VHAL_CANMsgInvalidEBC1_flg>"
  CANMsgInvalidEBC1/1 -> not6/1
  not6/1 -> bus_creator/6  "VINP_CANMsgValidEBC1_flg"
  bus_selector/7 -> CANMsgInvalidEBC2/1  "<VHAL_CANMsgInvalidEBC2_flg>"
  CANMsgInvalidEBC2/1 -> not7/1
  not7/1 -> bus_creator/7  "VINP_CANMsgValidEBC2_flg"
  bus_selector/8 -> CANMsgInvalidEBC5/1  "<VHAL_CANMsgInvalidEBC5_flg>"
  CANMsgInvalidEBC5/1 -> not8/1
  not8/1 -> bus_creator/8  "VINP_CANMsgValidEBC5_flg"
  bus_selector/9 -> CANMsgInvalidECASDM1/1  "<VHAL_CANMsgInvalidECASDM1_flg>"
  CANMsgInvalidECASDM1/1 -> not9/1
  not9/1 -> bus_creator/9  "VINP_CANMsgValidECASDM1_flg"
  bus_selector/10 -> CANMsgInvalidEMC1EM1/1  "<VHAL_CANMsgInvalidEMC1EM1_flg>"
  CANMsgInvalidEMC1EM1/1 -> not10/1
  not10/1 -> bus_creator/10  "VINP_CANMsgValidEMC1EM1_flg"
  bus_selector/11 -> CANMsgInvalidHRW/1  "<VHAL_CANMsgInvalidHRW_flg>"
  CANMsgInvalidHRW/1 -> not11/1
  not11/1 -> bus_creator/11  "VINP_CANMsgValidHRW_flg"
  bus_selector/12 -> CANMsgInvalidTC1/1  "<VHAL_CANMsgInvalidTC1_flg>"
  CANMsgInvalidTC1/1 -> not12/1
  not12/1 -> bus_creator/12  "VINP_CANMsgValidTC1_flg"
  [BHAL_outputs] -> bus_selector/1
  bus_creator/1 -> inp_CanValid_bus/1

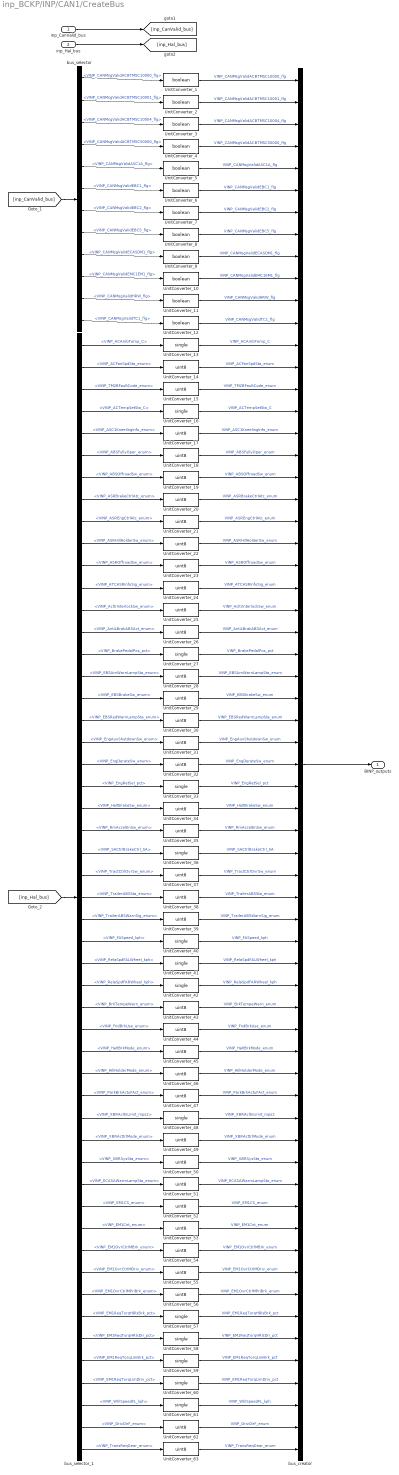
== system inp_BCKP/INP/CAN1/CreateBus ==
  inp_CanValid_bus : Inport
  inp_Hal_bus : Inport  Port=2
  UnitConverter_{1..12} (12 alike) : DataTypeConversion  OutDataTypeStr=boolean
  UnitConverter_{13,16,27,33,36,40..42,48,57..61} (14 alike) : DataTypeConversion  OutDataTypeStr=single
  UnitConverter_{14..15,17..26,28..32,34..35,37..39,43..47,49..56,62..63} (37 alike) : DataTypeConversion  OutDataTypeStr=uint8
  bus_creator : BusCreator  Inputs=63  OutDataTypeStr=Bus: BINP_CAN1_outputs  NonVirtualBus=on
  bus_selector : BusSelector  OutputSignals=VINP_CANMsgValidACBTMSC10000_flg,VINP_CANMsgValidACBTMSC10001_flg,VINP_CANMsgValidACBTMSC10004_flg,VINP_CANMsgValidACBTMSC50000_flg,VINP_CANMsgValidASC1A_flg,VINP_CANMsgValidEBC1_flg,VINP_CANMsgValidEBC2_flg,VINP_CANMsgValidEBC5_flg,VINP_CANMsgValidECASDM1_flg,VINP_CANMsgValidEMC1EM1_flg,VINP_CANMsgValidHRW_flg,VINP_CANMsgValidTC1_flg
  bus_selector_1 : BusSelector  OutputSignals=VINP_ACAmbTemp_C,VINP_ACFanSpdSta_enum,VINP_TM2BFaultCode_enum,VINP_ACTempSetSta_C,VINP_ASC1KneelingInfo_enum,VINP_ABSFullyOper_enum,VINP_ABSOffroadSw_enum,VINP_ASRBrakeCtrlAtc_enum,VINP_ASREngCtrlAtc_enum,VINP_ASRHillHolderSw_enum,VINP_ASROffroadSw_enum,VINP_ATCASRInfoSig_enum,VINP_AcltrInterlockSw_enum,VINP_AntiLBrakABSAct_enum,VINP_BrakePedalPos_pct,VINP_EBSAmWarnLampSta_enum,VINP_EBSBrakeSw_enum,VINP_EBSRedWarnLampSta_enum,VINP_EngAuxShutdownSw_enum,VINP_EngDerateSw_enum,VINP_EngRetSel_pct,VINP_HaltBrakeSw_enum,VINP_RmAccelEnSw_enum,VINP_SACtrlBrakeCtrl_SA,VINP_TractCtrlOvrSw_enum,VINP_TrailerABSSta_enum,VINP_TrailerABSWarnSig_enum,VINP_FASpeed_kph,VINP_RelaSpdFALWheel_kph,VINP_RelaSpdFARWheel_kph,VINP_BrkTempeWarn_enum,VINP_FndBrkUse_enum,VINP_HaltBrkMode_enum,VINP_HillHolderMode_enum,VINP_ParkBrkActuFAct_enum,VINP_XBRAcltnLimit_mps2,VINP_XBRActtrlMode_enum,VINP_XBRSysSta_enum,VINP_ECASAWarmLampSta_enum,VINP_EM1CS_enum,VINP_EM1Cnt_enum,VINP_EM1OvrCtrlMBrk_enum,VINP_EM1OvrCtrlMDriv_enum,VINP_EM1OvrCtrlMPriBrk_enum,VINP_EM1ReqTorqHRlsBrk_pct,VINP_EM1ReqTorqHRlsDri_pct,VINP_EM1ReqTorqLimBrk_pct,VINP_EM1ReqTorqLimDriv_pct,VINP_WhlSpeedFL_kph,VINP_DrivDirF_enum,VINP_TransReqGear_enum
  BINP_outputs : Outport
  wires:
  inp_CanValid_bus/1 -> [inp_CanValid_bus]
  inp_Hal_bus/1 -> [inp_Hal_bus]
  bus_selector/1 -> UnitConverter_1/1  "<VINP_CANMsgValidACBTMSC10000_flg>"
  UnitConverter_1/1 -> bus_creator/1  "VINP_CANMsgValidACBTMSC10000_flg"
  bus_selector/2 -> UnitConverter_2/1  "<VINP_CANMsgValidACBTMSC10001_flg>"
  UnitConverter_2/1 -> bus_creator/2  "VINP_CANMsgValidACBTMSC10001_flg"
  bus_selector/3 -> UnitConverter_3/1  "<VINP_CANMsgValidACBTMSC10004_flg>"
  UnitConverter_3/1 -> bus_creator/3  "VINP_CANMsgValidACBTMSC10004_flg"
  bus_selector/4 -> UnitConverter_4/1  "<VINP_CANMsgValidACBTMSC50000_flg>"
  UnitConverter_4/1 -> bus_creator/4  "VINP_CANMsgValidACBTMSC50000_flg"
  bus_selector/5 -> UnitConverter_5/1  "<VINP_CANMsgValidASC1A_flg>"
  UnitConverter_5/1 -> bus_creator/5  "VINP_CANMsgValidASC1A_flg"
  bus_selector/6 -> UnitConverter_6/1  "<VINP_CANMsgValidEBC1_flg>"
  UnitConverter_6/1 -> bus_creator/6  "VINP_CANMsgValidEBC1_flg"
  bus_selector/7 -> UnitConverter_7/1  "<VINP_CANMsgValidEBC2_flg>"
  UnitConverter_7/1 -> bus_creator/7  "VINP_CANMsgValidEBC2_flg"
  bus_selector/8 -> UnitConverter_8/1  "<VINP_CANMsgValidEBC5_flg>"
  UnitConverter_8/1 -> bus_creator/8  "VINP_CANMsgValidEBC5_flg"
  bus_selector/9 -> UnitConverter_9/1  "<VINP_CANMsgValidECASDM1_flg>"
  UnitConverter_9/1 -> bus_creator/9  "VINP_CANMsgValidECASDM1_flg"
  bus_selector/10 -> UnitConverter_10/1  "<VINP_CANMsgValidEMC1EM1_flg>"
  UnitConverter_10/1 -> bus_creator/10  "VINP_CANMsgValidEMC1EM1_flg"
  bus_selector/11 -> UnitConverter_11/1  "<VINP_CANMsgValidHRW_flg>"
  UnitConverter_11/1 -> bus_creator/11  "VINP_CANMsgValidHRW_flg"
  bus_selector/12 -> UnitConverter_12/1  "<VINP_CANMsgValidTC1_flg>"
  UnitConverter_12/1 -> bus_creator/12  "VINP_CANMsgValidTC1_flg"
  bus_selector_1/1 -> UnitConverter_13/1  "<VINP_ACAmbTemp_C>"
  UnitConverter_13/1 -> bus_creator/13  "VINP_ACAmbTemp_C"
  bus_selector_1/2 -> UnitConverter_14/1  "<VINP_ACFanSpdSta_enum>"
  UnitConverter_14/1 -> bus_creator/14  "VINP_ACFanSpdSta_enum"
  bus_selector_1/3 -> UnitConverter_15/1  "<VINP_TM2BFaultCode_enum>"
  UnitConverter_15/1 -> bus_creator/15  "VINP_TM2BFaultCode_enum"
  bus_selector_1/4 -> UnitConverter_16/1  "<VINP_ACTempSetSta_C>"
  UnitConverter_16/1 -> bus_creator/16  "VINP_ACTempSetSta_C"
  bus_selector_1/5 -> UnitConverter_17/1  "<VINP_ASC1KneelingInfo_enum>"
  UnitConverter_17/1 -> bus_creator/17  "VINP_ASC1KneelingInfo_enum"
  bus_selector_1/6 -> UnitConverter_18/1  "<VINP_ABSFullyOper_enum>"
  UnitConverter_18/1 -> bus_creator/18  "VINP_ABSFullyOper_enum"
  bus_selector_1/7 -> UnitConverter_19/1  "<VINP_ABSOffroadSw_enum>"
  UnitConverter_19/1 -> bus_creator/19  "VINP_ABSOffroadSw_enum"
  bus_selector_1/8 -> UnitConverter_20/1  "<VINP_ASRBrakeCtrlAtc_enum>"
  UnitConverter_20/1 -> bus_creator/20  "VINP_ASRBrakeCtrlAtc_enum"
  bus_selector_1/9 -> UnitConverter_21/1  "<VINP_ASREngCtrlAtc_enum>"
  UnitConverter_21/1 -> bus_creator/21  "VINP_ASREngCtrlAtc_enum"
  bus_selector_1/10 -> UnitConverter_22/1  "<VINP_ASRHillHolderSw_enum>"
  UnitConverter_22/1 -> bus_creator/22  "VINP_ASRHillHolderSw_enum"
  bus_selector_1/11 -> UnitConverter_23/1  "<VINP_ASROffroadSw_enum>"
  UnitConverter_23/1 -> bus_creator/23  "VINP_ASROffroadSw_enum"
  bus_selector_1/12 -> UnitConverter_24/1  "<VINP_ATCASRInfoSig_enum>"
  UnitConverter_24/1 -> bus_creator/24  "VINP_ATCASRInfoSig_enum"
  bus_selector_1/13 -> UnitConverter_25/1  "<VINP_AcltrInterlockSw_enum>"
  UnitConverter_25/1 -> bus_creator/25  "VINP_AcltrInterlockSw_enum"
  bus_selector_1/14 -> UnitConverter_26/1  "<VINP_AntiLBrakABSAct_enum>"
  UnitConverter_26/1 -> bus_creator/26  "VINP_AntiLBrakABSAct_enum"
  bus_selector_1/15 -> UnitConverter_27/1  "<VINP_BrakePedalPos_pct>"
  UnitConverter_27/1 -> bus_creator/27  "VINP_BrakePedalPos_pct"
  bus_selector_1/16 -> UnitConverter_28/1  "<VINP_EBSAmWarnLampSta_enum>"
  UnitConverter_28/1 -> bus_creator/28  "VINP_EBSAmWarnLampSta_enum"
  bus_selector_1/17 -> UnitConverter_29/1  "<VINP_EBSBrakeSw_enum>"
  UnitConverter_29/1 -> bus_creator/29  "VINP_EBSBrakeSw_enum"
  bus_selector_1/18 -> UnitConverter_30/1  "<VINP_EBSRedWarnLampSta_enum>"
  UnitConverter_30/1 -> bus_creator/30  "VINP_EBSRedWarnLampSta_enum"
  bus_selector_1/19 -> UnitConverter_31/1  "<VINP_EngAuxShutdownSw_enum>"
  UnitConverter_31/1 -> bus_creator/31  "VINP_EngAuxShutdownSw_enum"
  bus_selector_1/20 -> UnitConverter_32/1  "<VINP_EngDerateSw_enum>"
  UnitConverter_32/1 -> bus_creator/32  "VINP_EngDerateSw_enum"
  bus_selector_1/21 -> UnitConverter_33/1  "<VINP_EngRetSel_pct>"
  UnitConverter_33/1 -> bus_creator/33  "VINP_EngRetSel_pct"
  bus_selector_1/22 -> UnitConverter_34/1  "<VINP_HaltBrakeSw_enum>"
  UnitConverter_34/1 -> bus_creator/34  "VINP_HaltBrakeSw_enum"
  bus_selector_1/23 -> UnitConverter_35/1  "<VINP_RmAccelEnSw_enum>"
  UnitConverter_35/1 -> bus_creator/35  "VINP_RmAccelEnSw_enum"
  bus_selector_1/24 -> UnitConverter_36/1  "<VINP_SACtrlBrakeCtrl_SA>"
  UnitConverter_36/1 -> bus_creator/36  "VINP_SACtrlBrakeCtrl_SA"
  bus_selector_1/25 -> UnitConverter_37/1  "<VINP_TractCtrlOvrSw_enum>"
  UnitConverter_37/1 -> bus_creator/37  "VINP_TractCtrlOvrSw_enum"
  bus_selector_1/26 -> UnitConverter_38/1  "<VINP_TrailerABSSta_enum>"
  UnitConverter_38/1 -> bus_creator/38  "VINP_TrailerABSSta_enum"
  bus_selector_1/27 -> UnitConverter_39/1  "<VINP_TrailerABSWarnSig_enum>"
  UnitConverter_39/1 -> bus_creator/39  "VINP_TrailerABSWarnSig_enum"
  bus_selector_1/28 -> UnitConverter_40/1  "<VINP_FASpeed_kph>"
  UnitConverter_40/1 -> bus_creator/40  "VINP_FASpeed_kph"
  bus_selector_1/29 -> UnitConverter_41/1  "<VINP_RelaSpdFALWheel_kph>"
  UnitConverter_41/1 -> bus_creator/41  "VINP_RelaSpdFALWheel_kph"
  bus_selector_1/30 -> UnitConverter_42/1  "<VINP_RelaSpdFARWheel_kph>"
  UnitConverter_42/1 -> bus_creator/42  "VINP_RelaSpdFARWheel_kph"
  bus_selector_1/31 -> UnitConverter_43/1  "<VINP_BrkTempeWarn_enum>"
  UnitConverter_43/1 -> bus_creator/43  "VINP_BrkTempeWarn_enum"
  bus_selector_1/32 -> UnitConverter_44/1  "<VINP_FndBrkUse_enum>"
  UnitConverter_44/1 -> bus_creator/44  "VINP_FndBrkUse_enum"
  bus_selector_1/33 -> UnitConverter_45/1  "<VINP_HaltBrkMode_enum>"
  UnitConverter_45/1 -> bus_creator/45  "VINP_HaltBrkMode_enum"
  bus_selector_1/34 -> UnitConverter_46/1  "<VINP_HillHolderMode_enum>"
  UnitConverter_46/1 -> bus_creator/46  "VINP_HillHolderMode_enum"
  bus_selector_1/35 -> UnitConverter_47/1  "<VINP_ParkBrkActuFAct_enum>"
  UnitConverter_47/1 -> bus_creator/47  "VINP_ParkBrkActuFAct_enum"
  bus_selector_1/36 -> UnitConverter_48/1  "<VINP_XBRAcltnLimit_mps2>"
  UnitConverter_48/1 -> bus_creator/48  "VINP_XBRAcltnLimit_mps2"
  bus_selector_1/37 -> UnitConverter_49/1  "<VINP_XBRActtrlMode_enum>"
  UnitConverter_49/1 -> bus_creator/49  "VINP_XBRActtrlMode_enum"
  bus_selector_1/38 -> UnitConverter_50/1  "<VINP_XBRSysSta_enum>"
  UnitConverter_50/1 -> bus_creator/50  "VINP_XBRSysSta_enum"
  bus_selector_1/39 -> UnitConverter_51/1  "<VINP_ECASAWarmLampSta_enum>"
  UnitConverter_51/1 -> bus_creator/51  "VINP_ECASAWarmLampSta_enum"
  bus_selector_1/40 -> UnitConverter_52/1  "<VINP_EM1CS_enum>"
  UnitConverter_52/1 -> bus_creator/52  "VINP_EM1CS_enum"
  bus_selector_1/41 -> UnitConverter_53/1  "<VINP_EM1Cnt_enum>"
  UnitConverter_53/1 -> bus_creator/53  "VINP_EM1Cnt_enum"
  bus_selector_1/42 -> UnitConverter_54/1  "<VINP_EM1OvrCtrlMBrk_enum>"
  UnitConverter_54/1 -> bus_creator/54  "VINP_EM1OvrCtrlMBrk_enum"
  bus_selector_1/43 -> UnitConverter_55/1  "<VINP_EM1OvrCtrlMDriv_enum>"
  UnitConverter_55/1 -> bus_creator/55  "VINP_EM1OvrCtrlMDriv_enum"
  bus_selector_1/44 -> UnitConverter_56/1  "<VINP_EM1OvrCtrlMPriBrk_enum>"
  UnitConverter_56/1 -> bus_creator/56  "VINP_EM1OvrCtrlMPriBrk_enum"
  bus_selector_1/45 -> UnitConverter_57/1  "<VINP_EM1ReqTorqHRlsBrk_pct>"
  UnitConverter_57/1 -> bus_creator/57  "VINP_EM1ReqTorqHRlsBrk_pct"
  bus_selector_1/46 -> UnitConverter_58/1  "<VINP_EM1ReqTorqHRlsDri_pct>"
  UnitConverter_58/1 -> bus_creator/58  "VINP_EM1ReqTorqHRlsDri_pct"
  bus_selector_1/47 -> UnitConverter_59/1  "<VINP_EM1ReqTorqLimBrk_pct>"
  UnitConverter_59/1 -> bus_creator/59  "VINP_EM1ReqTorqLimBrk_pct"
  bus_selector_1/48 -> UnitConverter_60/1  "<VINP_EM1ReqTorqLimDriv_pct>"
  UnitConverter_60/1 -> bus_creator/60  "VINP_EM1ReqTorqLimDriv_pct"
  bus_selector_1/49 -> UnitConverter_61/1  "<VINP_WhlSpeedFL_kph>"
  UnitConverter_61/1 -> bus_creator/61  "VINP_WhlSpeedFL_kph"
  bus_selector_1/50 -> UnitConverter_62/1  "<VINP_DrivDirF_enum>"
  UnitConverter_62/1 -> bus_creator/62  "VINP_DrivDirF_enum"
  bus_selector_1/51 -> UnitConverter_63/1  "<VINP_TransReqGear_enum>"
  UnitConverter_63/1 -> bus_creator/63  "VINP_TransReqGear_enum"
  [inp_CanValid_bus] -> bus_selector/1
  [inp_Hal_bus] -> bus_selector_1/1
  bus_creator/1 -> BINP_outputs/1
